simulink model "dinamicaralik"  (R2023b)
settings: Solver=ode45  StartTime=0.0  StopTime=50  FixedStep=0.0001  RelTol=1e-3
InitFcn:
  | Kpz = 0.3 ;
  | KIz = 0;
  | 
  | bh = 0.010290;  % batan hacim m^3
  | m = 10.5     ;  % aracın kütlesi kg
  | g = 9.81     ;  % yer çekimi ivmesi
  | p = 1000     ; % kg / m^3 yogunluk
  | W = m*g      ;  % aracın agırlıgı N
  | B = p*g*bh   ;  % Kaldırma kuvveti  N
  | 
  | xg = 0 ; % rgid body frame e göre ağırlık merkzi kordinatları
  | yg = 0 ;
  | zg = 0.02 ;
  | 
  | Ix = 0.1011 ; % kg *  m ^2
  | Iy = 0.1159 ;
  | Iz = 0.1615 ;
  | 
  | thrustCoefficient = 50/21.5 ;
  | 
  | % Add mass parametreleri
  | Xu_dot = -5.5;   % Surge direction
  | Yv_dot = -12.7;  % Sway direction
  | Zw_dot = -14.57; % Heave direction
  | 
  | Kp_dot = -0.12;  % Roll moment
  | Mq_dot = -0.12;  % Pitch moment
  | Nr_dot = -0.12;  % Yaw moment
  | 
  | % Linear Damping Values (Doğrusal Sönümleme Katsayıları)
  | Xu = -4.03;   % Ns/m
  | Yv = -6.22;   % Ns/m
  | Zw = -5.18;   % Ns/m
  | Kp = -0.07;   % Ns/rad
  | Mq = -0.07;   % Ns/rad
  | Nr = -0.07;   % Ns/rad
  | 
  | % Quadratic Damping Values (Doğrusal Olmayan Sönümleme Katsayıları)
  | Xuu = -18.18;  % Ns^2/m^2
  | Yvv = -21.66;  % Ns^2/m^2
  | Zww = -36.99;  % Ns^2/m^2
  | Kpp = -1.55;   % Ns^2/rad^2
  | Mqq = -1.55;   % Ns^2/rad^2
  | Nrr = -1.55;   % Ns^2/rad^2
undefined symbols (not defined in the file or in its folder): smiData, X, Y, Z
libraries: slpidlib x41, nesl_utility x14, sm_lib x12
(part 1 of 7)
settings Model: Creator=Yaser  LastModifiedBy=User

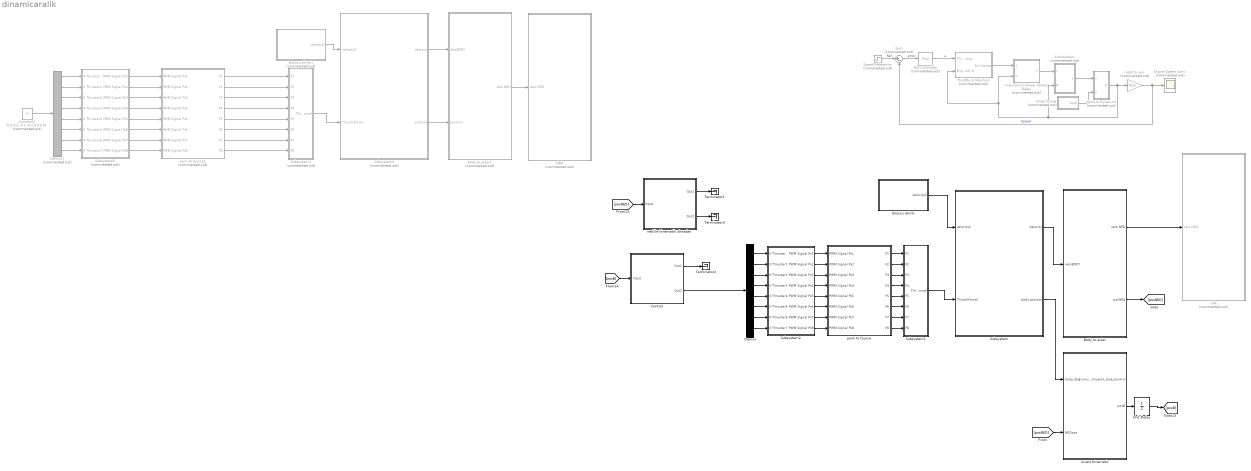
== system dinamicaralik ==
  Body to euler : Subsystem
  Body to euler1 : Subsystem  Commented=on
  Bozucu akıntı : Subsystem
  Bozucu akıntı1 : Subsystem  Commented=on
  Combustion : Subsystem  Commented=on
      settings: RTWMemSecFuncInitTerm=Default  RTWMemSecFuncExecute=Default  RTWMemSecDataConstants=Default  RTWMemSecDataInternal=Default  RTWMemSecDataParameters=Default
  Constant1 : Constant  Commented=on  Value=[0.2 0.2 -0.2 -0.2 0 0 0 0]  VectorParams1D=off
  Control : Subsystem
  Demux : Demux  Outputs=8
  Demux1 : Demux  Commented=on  Outputs=8
  Drag Torque : Subsystem  Commented=on
      settings: RTWMemSecFuncInitTerm=Default  RTWMemSecFuncExecute=Default  RTWMemSecDataConstants=Default  RTWMemSecDataInternal=Default  RTWMemSecDataParameters=Default
  Engine Speed (rpm) : Scope  Commented=on
  Induction to Power Stroke Delay : Subsystem  Commented=on
      settings: RTWMemSecFuncInitTerm=Default  RTWMemSecFuncExecute=Default  RTWMemSecDataConstants=Default  RTWMemSecDataInternal=Default  RTWMemSecDataParameters=Default
  Invers Kinematic : Subsystem
  PID Controller : slpidlib/PID Controller  Commented=on  Controller=PI  Form=Parallel  TimeDomain=Continuous-time  UseExternalTs=off  SampleTime=1  IntegratorMethod=Forward Euler  FilterMethod=Forward Euler  ControllerParametersSource=internal  P=1  I=1  UseKiTs=off  D=0  N=100  UseFilter=on  TunerSelectOption=Transfer Function Based (PID Tuner App)  ZeroCross=off  InitialConditionSource=internal  InitialConditionForIntegrator=8.9768  InitialConditionForFilter=0  DifferentiatorICPrevScaledInput=0  ExternalReset=none  TrackingMode=off  Kt=1  LimitOutput=off  SatLimitsSource=internal  UpperSaturationLimit=inf  LowerSaturationLimit=-inf  LinearizeAsGain=off  AntiWindupMode=none  Kb=1  LimitIntegrator=off  UpperIntegratorSaturationLimit=inf  LowerIntegratorSaturationLimit=-inf  POutMin=[ ]  POutMax=[ ]  IOutMin=[ ]  IOutMax=[ ]  DOutMin=[ ]  DOutMax=[ ]  NOutMin=[ ]  NOutMax=[ ]  SumOutMin=[ ]  SumOutMax=[ ]  SaturationOutMin=[ ]  SaturationOutMax=[ ]  PParamMin=[ ]  PParamMax=[ ]  IParamMin=[ ]  IParamMax=[ ]  DParamMin=[ ]  DParamMax=[ ]  NParamMin=[ ]  NParamMax=[ ]  KbParamMin=[ ]  KbParamMax=[ ]  KtParamMin=[ ]  KtParamMax=[ ]  KbOutMin=[ ]  KbOutMax=[ ]  KtOutMin=[ ]  KtOutMax=[ ]  IntegratorOutMin=[ ]  IntegratorOutMax=[ ]  FilterOutMin=[ ]  FilterOutMax=[ ]  SumI1OutMin=[ ]  SumI1OutMax=[ ]  SumI2OutMin=[ ]  SumI2OutMax=[ ]  SumI3OutMin=[ ]  SumI3OutMax=[ ]  SumI4OutMin=[]  SumI4OutMax=[]  SumDOutMin=[ ]  SumDOutMax=[ ]  DifferentiatorOutMin=[]  DifferentiatorOutMax=[]  FilterDiffOutCoefMin=[]  FilterDiffOutCoefMax=[]  ReciprocalOutMin=[]  ReciprocalOutMax=[]  SumDenOutMin=[]  SumDenOutMax=[]  SumNumOutMin=[]  SumNumOutMax=[]  DivideOutMin=[]  DivideOutMax=[]  UdiffTsProdOutMin=[]  UdiffTsProdOutMax=[]  NTsProdOutMin=[]  NTsProdOutMax=[]  UintegralTsProdOutMin=[]  UintegralTsProdOutMax=[]  UngainTsProdOutMin=[]  UngainTsProdOutMax=[]  ClampingZeroOutDataTypeStr=Inherit: Inherit via back propagation  ClampingZeroOutMin=[]  ClampingZeroOutMax=[]  FilterDenConstantOutDataTypeStr=Inherit: Inherit via back propagation  FilterDenConstantOutMin=[]  FilterDenConstantOutMax=[]  PCopyOutDataTypeStr=Inherit: Inherit via back propagation  PCopyOutMin=[]  PCopyOutMax=[]  NCopyOutDataTypeStr=Inherit: Inherit via back propagation  NCopyOutMin=[]  NCopyOutMax=[]  IntegratorContinuousStateAttributes=''  IntegratorStateMustResolveToSignalObject=off  IntegratorRTWStateStorageClass=Auto  FilterContinuousStateAttributes=''  FilterStateMustResolveToSignalObject=off  FilterRTWStateStorageClass=Auto  ParallelPVariant=InternalParameters  IdealPVariant=Disabled  IVariant=InternalParameters  DVariant=Disabled  IntegratorVariant=Continuous  SatVariant=Disabled  AWVariant=Passthrough  PCopyVariant=Disabled  TRVariant=Disabled  FdbkBlocksVariant=Forward  IdealPFdbkVariant=Disabled  SatFdbkVariant=Disabled  DerivativeFilterVariant=Disabled  NVariant=Disabled  NCopyVariant=Disabled_SignalSpec  FilterICVariant=Disabled  IntegratorICVariant=InternalICs  ExternalResetVariant=Disabled  TRSumVariant=Passthrough  SumFdbkVariant=Disabled  SumVariant=Sum_PI  TsampFilterVariant=InternalTs  TsampNgainVariant=Passthrough  TsampIntegralVariant=Disabled_SignalSpec  ExternalSaturationOutDataTypeStr=Inherit: Same as second input
  Speed Reference : Step  Commented=on  Time=2  Before=2000  After=3000  SampleTime=0
  Subsystem : Subsystem
  Subsystem1 : Subsystem
  Subsystem2 : Subsystem
  Subsystem3 : Subsystem  Commented=on
  Subsystem4 : Subsystem  Commented=on
  Subsystem5 : Subsystem  Commented=on
  Sum : Sum  Commented=on  Inputs=|+-
  SİM : Subsystem  Commented=on
  SİM1 : Subsystem  Commented=on
  Terminator1 : Terminator
  Terminator2 : Terminator
  Terminator3 : Terminator
  Throttle & Manifold : Subsystem  Commented=on
      settings: RTWMemSecFuncInitTerm=Default  RTWMemSecFuncExecute=Default  RTWMemSecDataConstants=Default  RTWMemSecDataInternal=Default  RTWMemSecDataParameters=Default
  Unit Delay : UnitDelay  SampleTime=0.01  HasFrameUpgradeWarning=on
  Vehicle Dynamics : Subsystem  Commented=on
      settings: RTWMemSecFuncInitTerm=Default  RTWMemSecFuncExecute=Default  RTWMemSecDataConstants=Default  RTWMemSecDataInternal=Default  RTWMemSecDataParameters=Default
  ned ile kinematik olmadan : Subsystem
  pwm to fource : Subsystem
  pwm to fource1 : Subsystem  Commented=on
  rad/s to rpm : Gain  Commented=on  Gain=30/pi  SaturateOnIntegerOverflow=on  OutDataTypeStr=Inherit: Same as input  ParamDataTypeStr=Inherit: Same as input
  wires:
  rad/s to rpm/1 -> Engine Speed (rpm)/1, Sum/2  "Speed"
  Throttle & Manifold/1(Air charge) -> Induction to Power Stroke Delay/1(Air charge)
  Induction to Power Stroke Delay/1(Air Charge) -> Combustion/1(Air Charge)
  Vehicle Dynamics/1(N) -> Combustion/2(N), Induction to Power Stroke Delay/2(N), Throttle & Manifold/2("Engine Speed, N"), rad/s to rpm/1
  Sum/1 -> PID Controller/1  "error"
  Combustion/1(Torque) -> Vehicle Dynamics/1(Teng)
  Drag Torque/1(Load) -> Vehicle Dynamics/2(Tload)
  PID Controller/1 -> Throttle & Manifold/1(Throttle Ang.)  "u"
  Speed Reference/1 -> Sum/1  "Ref"
  pwm to fource/4(F4) -> Subsystem1/4(F4)
  pwm to fource/3(F3) -> Subsystem1/3(F3)
  pwm to fource/2(F2) -> Subsystem1/2(F2)
  pwm to fource/1(F1) -> Subsystem1/1(F1)
  pwm to fource/5(F5) -> Subsystem1/5(F5)
  pwm to fource/6(F6) -> Subsystem1/6(F6)
  pwm to fource/7(F7) -> Subsystem1/7(F7)
  pwm to fource/8(F8) -> Subsystem1/8(F8)
  Subsystem2/1(PWM Signal Px1) -> pwm to fource/1(PWM Signal Px1)
  Subsystem2/2(PWM Signal Px2) -> pwm to fource/2(PWM Signal Px2)
  Subsystem2/3(PWM Signal Px3) -> pwm to fource/3(PWM Signal Px3)
  Subsystem2/4(PWM Signal Px4) -> pwm to fource/4(PWM Signal Px4)
  Subsystem2/5(PWM Signal Px5) -> pwm to fource/5(PWM Signal Px5)
  Subsystem2/6(PWM Signal Px6) -> pwm to fource/6(PWM Signal Px6)
  Subsystem2/7(PWM Signal Px7) -> pwm to fource/7(PWM Signal Px7)
  Subsystem2/8(PWM Signal Px8) -> pwm to fource/8(PWM Signal Px8)
  Bozucu akıntı/1(velocityC) -> Subsystem/1(velocityC)
  Subsystem/1(Velocity) -> Body to euler/1(veloBODY)
  Body to euler/1(velo NED) -> SİM/1(velo NED)
  Subsystem1/1(Thrust(Force)) -> Subsystem/2(Thrust(Force))
  Subsystem3/2(position) -> Body to euler1/2(position)
  Body to euler1/1(velo NED) -> SİM1/1(velo NED)
  Bozucu akıntı1/1(velocityC) -> Subsystem3/1(velocityC)
  Subsystem4/1(Thrust(Force)) -> Subsystem3/2(Thrust(Force))
  Subsystem5/6(PWM Signal Px6) -> pwm to fource1/6(PWM Signal Px6)
  Demux1/7 -> Subsystem5/7(X Thruster6)
  Subsystem5/5(PWM Signal Px5) -> pwm to fource1/5(PWM Signal Px5)
  Demux1/4 -> Subsystem5/4(X Thruster3)
  Subsystem5/7(PWM Signal Px7) -> pwm to fource1/7(PWM Signal Px7)
  Constant1/1 -> Demux1/1
  Demux1/2 -> Subsystem5/2(X Thruster1)
  Demux1/5 -> Subsystem5/5(X Thruster4)
  Demux1/1 -> Subsystem5/1(X Thruster)
  Subsystem5/8(PWM Signal Px8) -> pwm to fource1/8(PWM Signal Px8)
  Subsystem5/1(PWM Signal Px1) -> pwm to fource1/1(PWM Signal Px1)
  Demux1/3 -> Subsystem5/3(X Thruster2)
  pwm to fource1/6(F6) -> Subsystem4/6(F6)
  Subsystem3/1(Velocity) -> Body to euler1/1(veloBODY)
  Subsystem5/4(PWM Signal Px4) -> pwm to fource1/4(PWM Signal Px4)
  pwm to fource1/4(F4) -> Subsystem4/4(F4)
  Demux1/6 -> Subsystem5/6(X Thruster5)
  Subsystem5/2(PWM Signal Px2) -> pwm to fource1/2(PWM Signal Px2)
  pwm to fource1/5(F5) -> Subsystem4/5(F5)
  pwm to fource1/8(F8) -> Subsystem4/8(F8)
  pwm to fource1/2(F2) -> Subsystem4/2(F2)
  pwm to fource1/1(F1) -> Subsystem4/1(F1)
  Demux1/8 -> Subsystem5/8(X Thruster7)
  pwm to fource1/3(F3) -> Subsystem4/3(F3)
  pwm to fource1/7(F7) -> Subsystem4/7(F7)
  Subsystem5/3(PWM Signal Px3) -> pwm to fource1/3(PWM Signal Px3)
  Demux/1 -> Subsystem2/1(X Thruster)
  Demux/2 -> Subsystem2/2(X Thruster1)
  Demux/3 -> Subsystem2/3(X Thruster2)
  Demux/4 -> Subsystem2/4(X Thruster3)
  Demux/5 -> Subsystem2/5(X Thruster4)
  Demux/6 -> Subsystem2/6(X Thruster5)
  Demux/7 -> Subsystem2/7(X Thruster6)
  Demux/8 -> Subsystem2/8(X Thruster7)
  Body to euler/2(posNEd) -> [posNED]
  ned ile kinematik olmadan/1(Out1) -> Terminator1/1
  [posNED] -> ned ile kinematik olmadan/1(Input)
  Control/1(Out1) -> Terminator2/1
  Control/2(Out2) -> Demux/1
  [posB] -> Control/1(Input)
  ned ile kinematik olmadan/2(Out2) -> Terminator3/1
  Subsystem/2(body position) -> Invers Kinematic/1(body_doğrumudonuşum_diye_kontrol)
  [posNED] -> Invers Kinematic/2(NEDpos)
  Invers Kinematic/1(posB) -> Unit Delay/1
  Unit Delay/1 -> [posB]

== system dinamicaralik/Body to euler ==
  veloBODY : Inport
  Integrator : Integrator
  To Workspace : ToWorkspace  VariableName=pos  SaveFormat=Timeseries  SampleTime=-1
  euler transform : MATLAB Function  TreatAsAtomicUnit=on
  velo NED : Outport
  posNEd : Outport  Port=2
  wires:
  veloBODY/1 -> euler transform/1(veloB)
  euler transform/1(NEDvelo) -> Integrator/1, velo NED/1
  Integrator/1 -> To Workspace/1, posNEd/1

== system dinamicaralik/Body to euler1 ==
  veloBODY : Inport
  position : Inport  Port=2
  Integrator : Integrator
  To Workspace : ToWorkspace  VariableName=pos  SaveFormat=Timeseries  SampleTime=-1
  euler transform : MATLAB Function  TreatAsAtomicUnit=on
  velo NED : Outport
  wires:
  veloBODY/1 -> euler transform/1(veloB)
  euler transform/1(NEDvelo) -> Integrator/1, velo NED/1
  Integrator/1 -> To Workspace/1

== system dinamicaralik/Bozucu akıntı ==
  Constant : Constant  Value=[0 0 0 0 0 0 ]
  Constant1 : Constant  Commented=on  Value=[0 0 0 0 0 0 ]
  velocityC : Outport
  wires:
  Constant/1 -> velocityC/1

== system dinamicaralik/Bozucu akıntı1 ==
  Constant : Constant  Value=[0 0 0 0 0 0 ]
  Constant1 : Constant  Commented=on  Value=[0 0 0 0 0 0 ]
  velocityC : Outport
  wires:
  Constant/1 -> velocityC/1

== system dinamicaralik/Combustion ==
  note: Engine Torque
  Air Charge : Inport
  N : Inport  Port=2
  Mux : Mux
  Spark Advance : Constant  Value=15.0
  Stoichiometric Fuel : Gain  Gain=1/14.6  SaturateOnIntegerOverflow=on  OutDataTypeStr=Inherit: Same as input  ParamDataTypeStr=Inherit: Same as input
  Sum : Sum  InputSameDT=on  SaturateOnIntegerOverflow=on  OutDataTypeStr=Inherit: Same as first input
  Torque Gen : Fcn  Expr=-181.3 + 379.36*u[1] + 21.91*u[1]/u[2] - (0.85*u[1]*u[1])/(u[2]*u[2]) + 0.26*u[3] - 0.0028*u[3]*u[3]
  Torque Gen2 : Fcn  Expr=0.027*u[4] - 0.000107*u[4]*u[4] + 0.00048*u[4]*u[3] + 2.55*u[3]*u[1] - 0.05*u[3]*u[3]*u[1]
  Torque : Outport  InitialOutput=0  VectorParamsAs1DForOutWhenUnconnected=off
  wires:
  Stoichiometric Fuel/1 -> Mux/2
  Spark Advance/1 -> Mux/3
  N/1 -> Mux/4
  Air Charge/1 -> Stoichiometric Fuel/1, Mux/1
  Mux/1 -> Torque Gen/1, Torque Gen2/1
  Torque Gen2/1 -> Sum/2
  Torque Gen/1 -> Sum/1
  Sum/1 -> Torque/1

== system dinamicaralik/Control ==
  Input : Inport
  From : From  Commented=on  GotoTag=posNED
  divecont : Subsystem  Commented=on
  divecont1 : Subsystem
  Out1 : Outport
  Out2 : Outport  Port=2
  wires:
  Input/1 -> divecont1/1(Input)
  divecont1/1(Out1) -> Out2/1
  divecont/1(Out1) -> Out1/1
  From/1 -> divecont/1(In1)

== system dinamicaralik/Drag Torque ==
  note: Torque Disturbances
  Step : Step  Time=2  Before=25  After=25  SampleTime=0
  Step1 : Step  Time=8  After=0  SampleTime=0
  Sum1 : Sum  InputSameDT=on  SaturateOnIntegerOverflow=on  OutDataTypeStr=Inherit: Same as first input
  Load : Outport  InitialOutput=0  VectorParamsAs1DForOutWhenUnconnected=off
  wires:
  Step1/1 -> Sum1/2
  Step/1 -> Sum1/1
  Sum1/1 -> Load/1

== system dinamicaralik/Induction to Power Stroke Delay ==
  Air charge : Inport
  N : Inport  Port=2
  Constant2 : Constant  Value=pi
  Divide1 : Product  Inputs=/*
  dM/dt delay : VariableTransportDelay  MaximumDelay=10  InitialOutput=0.152  MaximumPoints=10240  TransDelayFeedthrough=on  PadeOrder=2
  Air Charge : Outport  VectorParamsAs1DForOutWhenUnconnected=off
  wires:
  dM/dt delay/1 -> Air Charge/1
  Constant2/1 -> Divide1/2
  N/1 -> Divide1/1
  Divide1/1 -> dM/dt delay/2
  Air charge/1 -> dM/dt delay/1

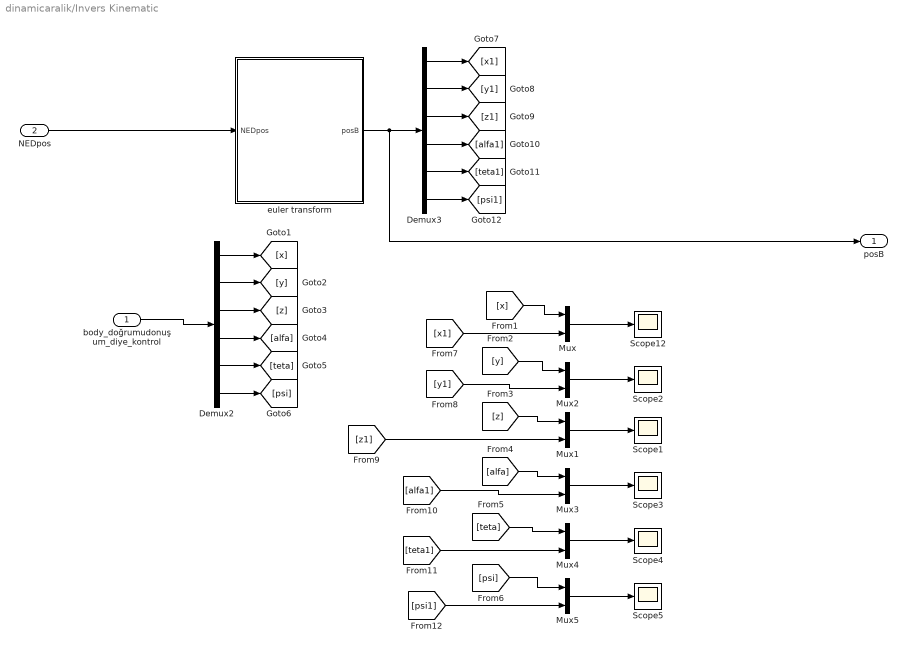
== system dinamicaralik/Invers Kinematic ==
  body_doğrumudonuşum_diye_kontrol : Inport
  NEDpos : Inport  Port=2
  Demux2 : Demux  Outputs=6
  Demux3 : Demux  Outputs=6
  Mux{,1..5} (6 alike) : Mux  Inputs=2
  Scope{1..5,12} (6 alike) : Scope
  euler transform : MATLAB Function  TreatAsAtomicUnit=on
  posB : Outport
  wires:
  [psi1] -> Mux5/2
  body_doğrumudonuşum_diye_kontrol/1 -> Demux2/1
  [x1] -> Mux/2
  Mux4/1 -> Scope4/1
  [z] -> Mux1/1
  euler transform/1(posB) -> posB/1, Demux3/1
  Demux3/1 -> [x1]
  Demux3/4 -> [alfa1]
  Demux3/5 -> [teta1]
  [z1] -> Mux1/2
  [y1] -> Mux2/2
  Mux3/1 -> Scope3/1
  [x] -> Mux/1
  Demux2/5 -> [teta]
  [psi] -> Mux5/1
  Demux3/6 -> [psi1]
  [alfa1] -> Mux3/2
  [teta1] -> Mux4/2
  [alfa] -> Mux3/1
  [teta] -> Mux4/1
  Mux2/1 -> Scope2/1
  Demux3/2 -> [y1]
  Demux2/1 -> [x]
  Mux1/1 -> Scope1/1
  [y] -> Mux2/1
  Demux3/3 -> [z1]
  Demux2/3 -> [z]
  Mux5/1 -> Scope5/1
  NEDpos/1 -> euler transform/1(NEDpos)
  Demux2/2 -> [y]
  Demux2/6 -> [psi]
  Mux/1 -> Scope12/1
  Demux2/4 -> [alfa]

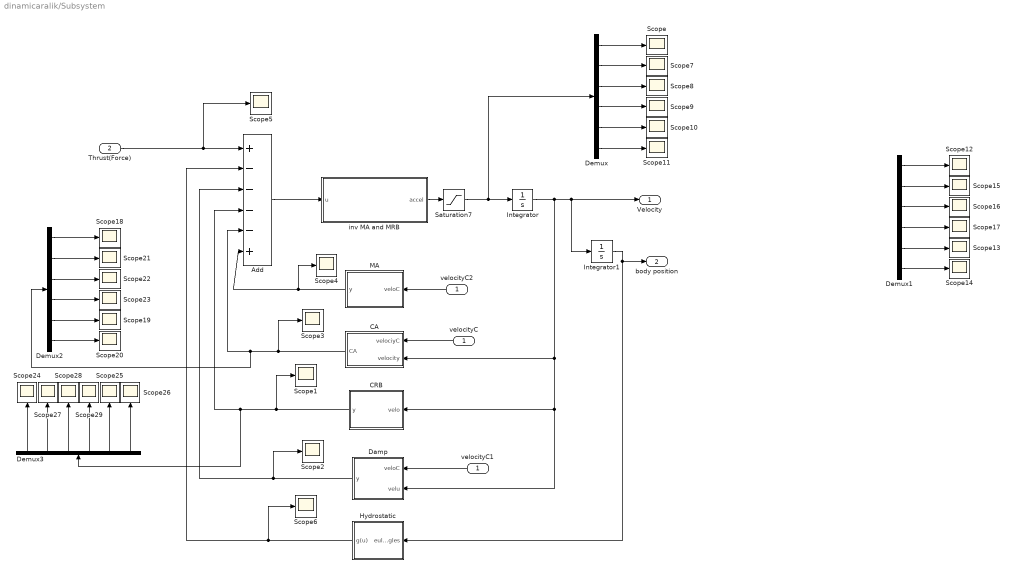
== system dinamicaralik/Subsystem ==
  velocityC : Inport
  Thrust(Force) : Inport  Port=2
  Add : Sum  Inputs=+----+
  CA : Subsystem
  CRB : Subsystem
  Damp : Subsystem
  Demux{,1..3} (4 alike) : Demux  Outputs=6
  Hydrostatic : Subsystem
  Integrator : Integrator
  Integrator1 : Integrator
  MA : Subsystem
  Saturation7 : Saturate  UpperLimit=1000  LowerLimit=-100
  Scope{,1..29} (30 alike) : Scope
  inv MA and MRB : Subsystem
  velocityC1 : InportShadow
  velocityC2 : InportShadow
  Velocity : Outport
  body position : Outport  Port=2
  wires:
  CA/1(CA) -> Scope3/1, Demux2/1, Add/5
  CRB/1(y) -> Scope1/1, Demux3/1, Add/4
  Integrator1/1 -> body position/1, Hydrostatic/1(euler angles)
  Add/1 -> inv MA and MRB/1(u)
  Integrator/1 -> Integrator1/1, Velocity/1, Damp/2(velu), CRB/1(velo), CA/2(velocity)
  Hydrostatic/1(g(u)) -> Scope6/1, Add/2
  Damp/1(y) -> Scope2/1, Add/3
  velocityC/1 -> CA/1(velociyC)
  velocityC1/1 -> Damp/1(veloC)
  velocityC2/1 -> MA/1(veloC)
  MA/1(y) -> Scope4/1, Add/6
  inv MA and MRB/1(accel) -> Saturation7/1
  Saturation7/1 -> Demux/1, Integrator/1
  Thrust(Force)/1 -> Scope5/1, Add/1
  Demux/1 -> Scope/1
  Demux/2 -> Scope7/1
  Demux/3 -> Scope8/1
  Demux/4 -> Scope9/1
  Demux/5 -> Scope10/1
  Demux/6 -> Scope11/1
  Demux1/1 -> Scope12/1
  Demux1/3 -> Scope16/1
  Demux1/6 -> Scope14/1
  Demux1/2 -> Scope15/1
  Demux1/4 -> Scope17/1
  Demux1/5 -> Scope13/1
  Demux2/1 -> Scope18/1
  Demux2/4 -> Scope23/1
  Demux2/2 -> Scope21/1
  Demux2/3 -> Scope22/1
  Demux2/5 -> Scope19/1
  Demux2/6 -> Scope20/1
  Demux3/5 -> Scope25/1
  Demux3/3 -> Scope28/1
  Demux3/2 -> Scope27/1
  Demux3/1 -> Scope24/1
  Demux3/4 -> Scope29/1
  Demux3/6 -> Scope26/1

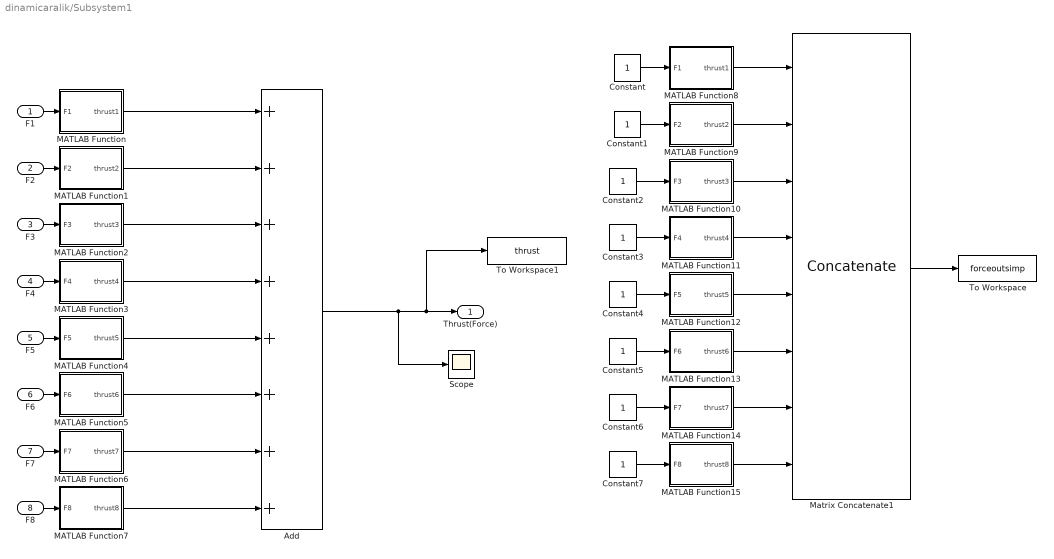
== system dinamicaralik/Subsystem1 ==
  F1 : Inport
  F2 : Inport  Port=2
  F3 : Inport  Port=3
  F4 : Inport  Port=4
  F5 : Inport  Port=5
  F6 : Inport  Port=6
  F7 : Inport  Port=7
  F8 : Inport  Port=8
  Add : Sum  Inputs=++++++++
  Constant{,1..7} (8 alike) : Constant
  MATLAB Function : MATLAB Function  TreatAsAtomicUnit=on
  MATLAB Function1 : MATLAB Function  TreatAsAtomicUnit=on
  MATLAB Function10 : MATLAB Function  TreatAsAtomicUnit=on
  MATLAB Function11 : MATLAB Function  TreatAsAtomicUnit=on
  MATLAB Function12 : MATLAB Function  TreatAsAtomicUnit=on
  MATLAB Function13 : MATLAB Function  TreatAsAtomicUnit=on
  MATLAB Function14 : MATLAB Function  TreatAsAtomicUnit=on
  MATLAB Function15 : MATLAB Function  TreatAsAtomicUnit=on
  MATLAB Function2 : MATLAB Function  TreatAsAtomicUnit=on
  MATLAB Function3 : MATLAB Function  TreatAsAtomicUnit=on
  MATLAB Function4 : MATLAB Function  TreatAsAtomicUnit=on
  MATLAB Function5 : MATLAB Function  TreatAsAtomicUnit=on
  MATLAB Function6 : MATLAB Function  TreatAsAtomicUnit=on
  MATLAB Function7 : MATLAB Function  TreatAsAtomicUnit=on
  MATLAB Function8 : MATLAB Function  TreatAsAtomicUnit=on
  MATLAB Function9 : MATLAB Function  TreatAsAtomicUnit=on
  Matrix Concatenate1 : Concatenate  NumInputs=8  Mode=Multidimensional array  ConcatenateDimension=2
  Scope : Scope
  To Workspace : ToWorkspace  VariableName=forceoutsimp  SaveFormat=Timeseries  SampleTime=-1
  To Workspace1 : ToWorkspace  VariableName=thrust  SaveFormat=Timeseries  SampleTime=-1
  Thrust(Force) : Outport
  wires:
  F1/1 -> MATLAB Function/1(F1)
  F4/1 -> MATLAB Function3/1(F4)
  F7/1 -> MATLAB Function6/1(F7)
  F3/1 -> MATLAB Function2/1(F3)
  F8/1 -> MATLAB Function7/1(F8)
  F5/1 -> MATLAB Function4/1(F5)
  F2/1 -> MATLAB Function1/1(F2)
  F6/1 -> MATLAB Function5/1(F6)
  MATLAB Function/1(thrust1) -> Add/1
  MATLAB Function1/1(thrust2) -> Add/2
  MATLAB Function3/1(thrust4) -> Add/4
  MATLAB Function4/1(thrust5) -> Add/5
  MATLAB Function5/1(thrust6) -> Add/6
  MATLAB Function6/1(thrust7) -> Add/7
  MATLAB Function7/1(thrust8) -> Add/8
  Add/1 -> Scope/1, To Workspace1/1, Thrust(Force)/1
  MATLAB Function2/1(thrust3) -> Add/3
  Constant7/1 -> MATLAB Function15/1(F8)
  Constant5/1 -> MATLAB Function13/1(F6)
  Constant2/1 -> MATLAB Function10/1(F3)
  Constant6/1 -> MATLAB Function14/1(F7)
  Constant/1 -> MATLAB Function8/1(F1)
  Constant4/1 -> MATLAB Function12/1(F5)
  Constant1/1 -> MATLAB Function9/1(F2)
  MATLAB Function14/1(thrust7) -> Matrix Concatenate1/7
  MATLAB Function9/1(thrust2) -> Matrix Concatenate1/2
  MATLAB Function13/1(thrust6) -> Matrix Concatenate1/6
  MATLAB Function8/1(thrust1) -> Matrix Concatenate1/1
  MATLAB Function10/1(thrust3) -> Matrix Concatenate1/3
  MATLAB Function11/1(thrust4) -> Matrix Concatenate1/4
  MATLAB Function15/1(thrust8) -> Matrix Concatenate1/8
  MATLAB Function12/1(thrust5) -> Matrix Concatenate1/5
  Constant3/1 -> MATLAB Function11/1(F4)
  Matrix Concatenate1/1 -> To Workspace/1

== system dinamicaralik/Subsystem2 ==
  X Thruster : Inport
  X Thruster1 : Inport  Port=2
  X Thruster2 : Inport  Port=3
  X Thruster3 : Inport  Port=4
  X Thruster4 : Inport  Port=5
  X Thruster5 : Inport  Port=6
  X Thruster6 : Inport  Port=7
  X Thruster7 : Inport  Port=8
  1-D Lookup Table{,1..7} (8 alike) : Lookup_n-D  NumberOfTableDimensions=1  BreakpointsForDimension1=[-1:0.01:1]  Table=1500 + 400 * ([-1:0.01:1])  InternalRulePriority=Speed  RndMeth=Simplest
  PWM Signal Px1 : Outport
  PWM Signal Px2 : Outport  Port=2
  PWM Signal Px3 : Outport  Port=3
  PWM Signal Px4 : Outport  Port=4
  PWM Signal Px5 : Outport  Port=5
  PWM Signal Px6 : Outport  Port=6
  PWM Signal Px7 : Outport  Port=7
  PWM Signal Px8 : Outport  Port=8
  wires:
  X Thruster2/1 -> 1-D Lookup Table2/1
  X Thruster5/1 -> 1-D Lookup Table5/1
  X Thruster/1 -> 1-D Lookup Table/1
  X Thruster6/1 -> 1-D Lookup Table6/1
  X Thruster4/1 -> 1-D Lookup Table4/1
  X Thruster1/1 -> 1-D Lookup Table1/1
  X Thruster3/1 -> 1-D Lookup Table3/1
  1-D Lookup Table1/1 -> PWM Signal Px2/1
  X Thruster7/1 -> 1-D Lookup Table7/1
  1-D Lookup Table/1 -> PWM Signal Px1/1
  1-D Lookup Table7/1 -> PWM Signal Px8/1
  1-D Lookup Table2/1 -> PWM Signal Px3/1
  1-D Lookup Table6/1 -> PWM Signal Px7/1
  1-D Lookup Table3/1 -> PWM Signal Px4/1
  1-D Lookup Table5/1 -> PWM Signal Px6/1
  1-D Lookup Table4/1 -> PWM Signal Px5/1

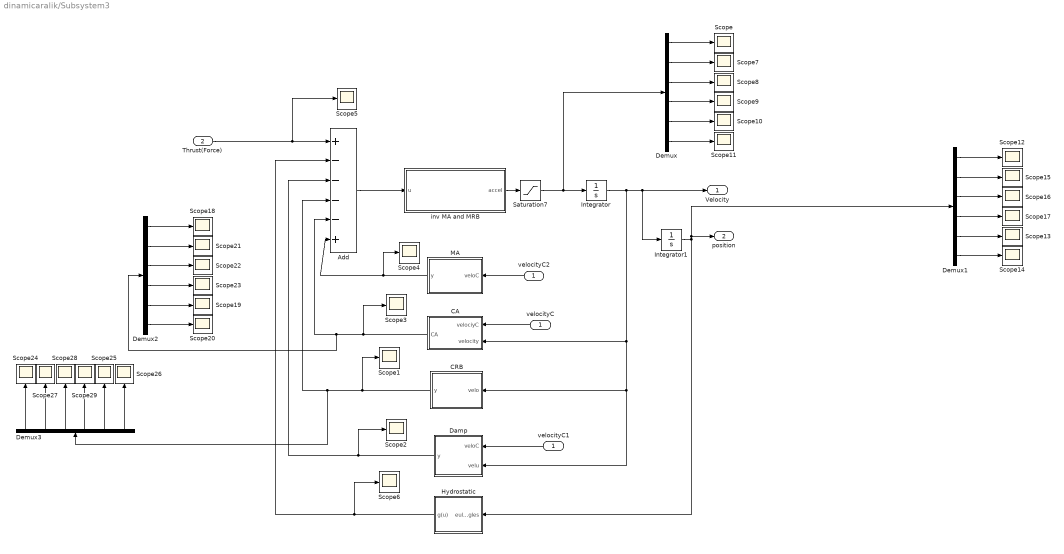
== system dinamicaralik/Subsystem3 ==
  velocityC : Inport
  Thrust(Force) : Inport  Port=2
  Add : Sum  Inputs=+----+
  CA : Subsystem
  CRB : Subsystem
  Damp : Subsystem
  Demux{,1..3} (4 alike) : Demux  Outputs=6
  Hydrostatic : Subsystem
  Integrator : Integrator
  Integrator1 : Integrator
  MA : Subsystem
  Saturation7 : Saturate  UpperLimit=1000  LowerLimit=-100
  Scope{,1..29} (30 alike) : Scope
  inv MA and MRB : Subsystem
  velocityC1 : InportShadow
  velocityC2 : InportShadow
  Velocity : Outport
  position : Outport  Port=2
  wires:
  CA/1(CA) -> Scope3/1, Demux2/1, Add/5
  CRB/1(y) -> Scope1/1, Demux3/1, Add/4
  Integrator1/1 -> Demux1/1, position/1, Hydrostatic/1(euler angles)
  Add/1 -> inv MA and MRB/1(u)
  Integrator/1 -> Integrator1/1, Velocity/1, Damp/2(velu), CRB/1(velo), CA/2(velocity)
  Hydrostatic/1(g(u)) -> Scope6/1, Add/2
  Damp/1(y) -> Scope2/1, Add/3
  velocityC/1 -> CA/1(velociyC)
  velocityC1/1 -> Damp/1(veloC)
  velocityC2/1 -> MA/1(veloC)
  MA/1(y) -> Scope4/1, Add/6
  inv MA and MRB/1(accel) -> Saturation7/1
  Saturation7/1 -> Demux/1, Integrator/1
  Thrust(Force)/1 -> Scope5/1, Add/1
  Demux/1 -> Scope/1
  Demux/2 -> Scope7/1
  Demux/3 -> Scope8/1
  Demux/4 -> Scope9/1
  Demux/5 -> Scope10/1
  Demux/6 -> Scope11/1
  Demux1/1 -> Scope12/1
  Demux1/3 -> Scope16/1
  Demux1/6 -> Scope14/1
  Demux1/2 -> Scope15/1
  Demux1/4 -> Scope17/1
  Demux1/5 -> Scope13/1
  Demux2/1 -> Scope18/1
  Demux2/4 -> Scope23/1
  Demux2/2 -> Scope21/1
  Demux2/3 -> Scope22/1
  Demux2/5 -> Scope19/1
  Demux2/6 -> Scope20/1
  Demux3/5 -> Scope25/1
  Demux3/3 -> Scope28/1
  Demux3/2 -> Scope27/1
  Demux3/1 -> Scope24/1
  Demux3/4 -> Scope29/1
  Demux3/6 -> Scope26/1

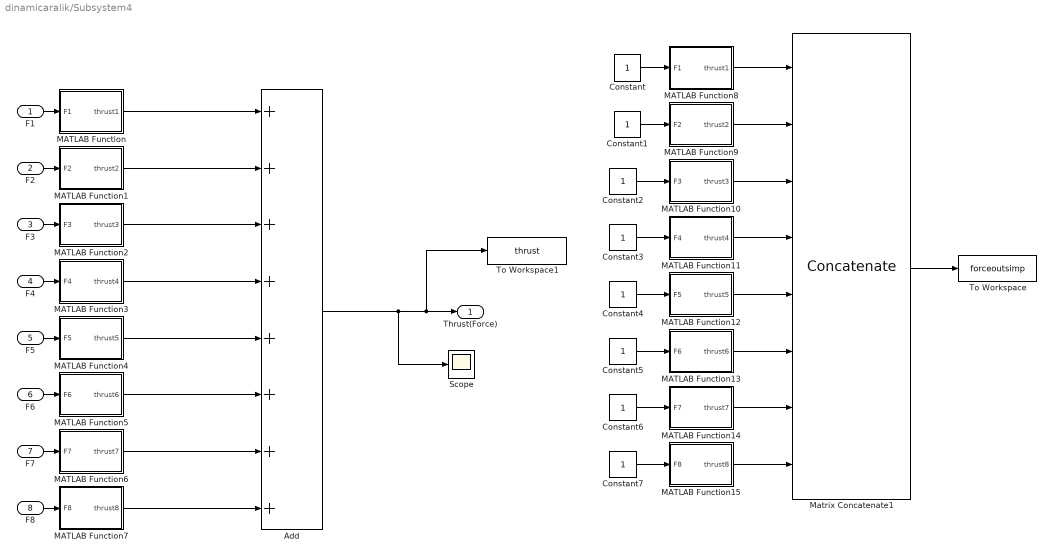
== system dinamicaralik/Subsystem4 ==
  F1 : Inport
  F2 : Inport  Port=2
  F3 : Inport  Port=3
  F4 : Inport  Port=4
  F5 : Inport  Port=5
  F6 : Inport  Port=6
  F7 : Inport  Port=7
  F8 : Inport  Port=8
  Add : Sum  Inputs=++++++++
  Constant{,1..7} (8 alike) : Constant
  MATLAB Function : MATLAB Function  TreatAsAtomicUnit=on
  MATLAB Function1 : MATLAB Function  TreatAsAtomicUnit=on
  MATLAB Function10 : MATLAB Function  TreatAsAtomicUnit=on
  MATLAB Function11 : MATLAB Function  TreatAsAtomicUnit=on
  MATLAB Function12 : MATLAB Function  TreatAsAtomicUnit=on
  MATLAB Function13 : MATLAB Function  TreatAsAtomicUnit=on
  MATLAB Function14 : MATLAB Function  TreatAsAtomicUnit=on
  MATLAB Function15 : MATLAB Function  TreatAsAtomicUnit=on
  MATLAB Function2 : MATLAB Function  TreatAsAtomicUnit=on
  MATLAB Function3 : MATLAB Function  TreatAsAtomicUnit=on
  MATLAB Function4 : MATLAB Function  TreatAsAtomicUnit=on
  MATLAB Function5 : MATLAB Function  TreatAsAtomicUnit=on
  MATLAB Function6 : MATLAB Function  TreatAsAtomicUnit=on
  MATLAB Function7 : MATLAB Function  TreatAsAtomicUnit=on
  MATLAB Function8 : MATLAB Function  TreatAsAtomicUnit=on
  MATLAB Function9 : MATLAB Function  TreatAsAtomicUnit=on
  Matrix Concatenate1 : Concatenate  NumInputs=8  Mode=Multidimensional array  ConcatenateDimension=2
  Scope : Scope
  To Workspace : ToWorkspace  VariableName=forceoutsimp  SaveFormat=Timeseries  SampleTime=-1
  To Workspace1 : ToWorkspace  VariableName=thrust  SaveFormat=Timeseries  SampleTime=-1
  Thrust(Force) : Outport
  wires:
  F1/1 -> MATLAB Function/1(F1)
  F4/1 -> MATLAB Function3/1(F4)
  F7/1 -> MATLAB Function6/1(F7)
  F3/1 -> MATLAB Function2/1(F3)
  F8/1 -> MATLAB Function7/1(F8)
  F5/1 -> MATLAB Function4/1(F5)
  F2/1 -> MATLAB Function1/1(F2)
  F6/1 -> MATLAB Function5/1(F6)
  MATLAB Function/1(thrust1) -> Add/1
  MATLAB Function1/1(thrust2) -> Add/2
  MATLAB Function3/1(thrust4) -> Add/4
  MATLAB Function4/1(thrust5) -> Add/5
  MATLAB Function5/1(thrust6) -> Add/6
  MATLAB Function6/1(thrust7) -> Add/7
  MATLAB Function7/1(thrust8) -> Add/8
  Add/1 -> Scope/1, To Workspace1/1, Thrust(Force)/1
  MATLAB Function2/1(thrust3) -> Add/3
  Constant7/1 -> MATLAB Function15/1(F8)
  Constant5/1 -> MATLAB Function13/1(F6)
  Constant2/1 -> MATLAB Function10/1(F3)
  Constant6/1 -> MATLAB Function14/1(F7)
  Constant/1 -> MATLAB Function8/1(F1)
  Constant4/1 -> MATLAB Function12/1(F5)
  Constant1/1 -> MATLAB Function9/1(F2)
  MATLAB Function14/1(thrust7) -> Matrix Concatenate1/7
  MATLAB Function9/1(thrust2) -> Matrix Concatenate1/2
  MATLAB Function13/1(thrust6) -> Matrix Concatenate1/6
  MATLAB Function8/1(thrust1) -> Matrix Concatenate1/1
  MATLAB Function10/1(thrust3) -> Matrix Concatenate1/3
  MATLAB Function11/1(thrust4) -> Matrix Concatenate1/4
  MATLAB Function15/1(thrust8) -> Matrix Concatenate1/8
  MATLAB Function12/1(thrust5) -> Matrix Concatenate1/5
  Constant3/1 -> MATLAB Function11/1(F4)
  Matrix Concatenate1/1 -> To Workspace/1

== system dinamicaralik/Subsystem5 ==
  X Thruster : Inport
  X Thruster1 : Inport  Port=2
  X Thruster2 : Inport  Port=3
  X Thruster3 : Inport  Port=4
  X Thruster4 : Inport  Port=5
  X Thruster5 : Inport  Port=6
  X Thruster6 : Inport  Port=7
  X Thruster7 : Inport  Port=8
  1-D Lookup Table{,1..7} (8 alike) : Lookup_n-D  NumberOfTableDimensions=1  BreakpointsForDimension1=[-1:0.01:1]  Table=1500 + 400 * ([-1:0.01:1])  InternalRulePriority=Speed  RndMeth=Simplest
  PWM Signal Px1 : Outport
  PWM Signal Px2 : Outport  Port=2
  PWM Signal Px3 : Outport  Port=3
  PWM Signal Px4 : Outport  Port=4
  PWM Signal Px5 : Outport  Port=5
  PWM Signal Px6 : Outport  Port=6
  PWM Signal Px7 : Outport  Port=7
  PWM Signal Px8 : Outport  Port=8
  wires:
  X Thruster2/1 -> 1-D Lookup Table2/1
  X Thruster5/1 -> 1-D Lookup Table5/1
  X Thruster/1 -> 1-D Lookup Table/1
  X Thruster6/1 -> 1-D Lookup Table6/1
  X Thruster4/1 -> 1-D Lookup Table4/1
  X Thruster1/1 -> 1-D Lookup Table1/1
  X Thruster3/1 -> 1-D Lookup Table3/1
  1-D Lookup Table1/1 -> PWM Signal Px2/1
  X Thruster7/1 -> 1-D Lookup Table7/1
  1-D Lookup Table/1 -> PWM Signal Px1/1
  1-D Lookup Table7/1 -> PWM Signal Px8/1
  1-D Lookup Table2/1 -> PWM Signal Px3/1
  1-D Lookup Table6/1 -> PWM Signal Px7/1
  1-D Lookup Table3/1 -> PWM Signal Px4/1
  1-D Lookup Table5/1 -> PWM Signal Px6/1
  1-D Lookup Table4/1 -> PWM Signal Px5/1

== system dinamicaralik/SİM ==
  velo NED : Inport
  6-DOF Joint : sm_lib/Joints/6-DOF Joint  JointMode=Normal  SenseConstraintForce=off  SenseConstraintForceX=off  SenseConstraintForceY=off  SenseConstraintForceZ=off  SenseConstraintTorque=off  SenseConstraintTorqueX=off  SenseConstraintTorqueY=off  SenseConstraintTorqueZ=off  SenseTotalForce=off  SenseTotalForceX=off  SenseTotalForceY=off  SenseTotalForceZ=off  SenseTotalTorque=off  SenseTotalTorqueX=off  SenseTotalTorqueY=off  SenseTotalTorqueZ=off  CompositeWrenchDir=FollowerOnBase  CompositeWrenchFrame=BaseFrame  PxEquilibriumPosition=0  PxEquilibriumPositionUnits=m  PxSpringStiffness=0  PxSpringStiffnessUnits=N/m  PxDampingCoefficient=0  PxDampingCoefficientUnits=N/(m/s)  PxTorqueActuationMode=ComputedTorque  PxMotionActuationMode=InputMotion  PxSensePosition=off  PxSenseVelocity=off  PxSenseAcceleration=off  PxSenseTorqueForce=off  PxSenseLowerLimitTorqueForce=off  PxSenseUpperLimitTorqueForce=off  PxLowerLimitSpecify=off  PxLowerLimitBound=-1  PxLowerLimitBoundUnits=m  PxLowerLimitStiffness=1e6  PxLowerLimitStiffnessUnits=N/m  PxLowerLimitDamping=1e3  PxLowerLimitDampingUnits=N/(m/s)  PxLowerLimitTransitionRegionWidth=1e-4  PxLowerLimitTransitionRegionWidthUnits=m  PxUpperLimitSpecify=off  PxUpperLimitBound=1  PxUpperLimitBoundUnits=m  PxUpperLimitStiffness=1e6  PxUpperLimitStiffnessUnits=N/m  PxUpperLimitDamping=1e3  PxUpperLimitDampingUnits=N/(m/s)  PxUpperLimitTransitionRegionWidth=1e-4  PxUpperLimitTransitionRegionWidthUnits=m  PxPositionTargetSpecify=off  PxPositionTargetPriority=High  PxPositionTargetValue=0  PxPositionTargetValueUnits=m  PxVelocityTargetSpecify=off  PxVelocityTargetPriority=High  PxVelocityTargetValue=0  PxVelocityTargetValueUnits=m/s  PyEquilibriumPosition=0  PyEquilibriumPositionUnits=m  PySpringStiffness=0  PySpringStiffnessUnits=N/m  PyDampingCoefficient=0  PyDampingCoefficientUnits=N/(m/s)  PyTorqueActuationMode=ComputedTorque  PyMotionActuationMode=InputMotion  PySensePosition=off  PySenseVelocity=off  PySenseAcceleration=off  PySenseTorqueForce=off  PySenseLowerLimitTorqueForce=off  PySenseUpperLimitTorqueForce=off  PyLowerLimitSpecify=off  PyLowerLimitBound=-1  PyLowerLimitBoundUnits=m  PyLowerLimitStiffness=1e6  PyLowerLimitStiffnessUnits=N/m  PyLowerLimitDamping=1e3  PyLowerLimitDampingUnits=N/(m/s)  PyLowerLimitTransitionRegionWidth=1e-4  PyLowerLimitTransitionRegionWidthUnits=m  PyUpperLimitSpecify=off  PyUpperLimitBound=1  PyUpperLimitBoundUnits=m  PyUpperLimitStiffness=1e6  PyUpperLimitStiffnessUnits=N/m  PyUpperLimitDamping=1e3  PyUpperLimitDampingUnits=N/(m/s)  PyUpperLimitTransitionRegionWidth=1e-4  PyUpperLimitTransitionRegionWidthUnits=m  PyPositionTargetSpecify=off  PyPositionTargetPriority=High  PyPositionTargetValue=0  PyPositionTargetValueUnits=m  PyVelocityTargetSpecify=off  PyVelocityTargetPriority=High  PyVelocityTargetValue=0  PyVelocityTargetValueUnits=m/s  PzEquilibriumPosition=0  PzEquilibriumPositionUnits=m  PzSpringStiffness=0  PzSpringStiffnessUnits=N/m  PzDampingCoefficient=0  PzDampingCoefficientUnits=N/(m/s)  PzTorqueActuationMode=ComputedTorque  PzMotionActuationMode=InputMotion  PzSensePosition=off  PzSenseVelocity=off  PzSenseAcceleration=off  PzSenseTorqueForce=off  PzSenseLowerLimitTorqueForce=off  PzSenseUpperLimitTorqueForce=off  PzLowerLimitSpecify=off  PzLowerLimitBound=-1  PzLowerLimitBoundUnits=m  PzLowerLimitStiffness=1e6  PzLowerLimitStiffnessUnits=N/m  PzLowerLimitDamping=1e3  PzLowerLimitDampingUnits=N/(m/s)  PzLowerLimitTransitionRegionWidth=1e-4  PzLowerLimitTransitionRegionWidthUnits=m  PzUpperLimitSpecify=off  PzUpperLimitBound=1  PzUpperLimitBoundUnits=m  PzUpperLimitStiffness=1e6  PzUpperLimitStiffnessUnits=N/m  PzUpperLimitDamping=1e3  PzUpperLimitDampingUnits=N/(m/s)  PzUpperLimitTransitionRegionWidth=1e-4  PzUpperLimitTransitionRegionWidthUnits=m  PzPositionTargetSpecify=off  PzPositionTargetPriority=High  PzPositionTargetValue=0  PzPositionTargetValueUnits=m  PzVelocityTargetSpecify=off  PzVelocityTargetPriority=High  PzVelocityTargetValue=0  PzVelocityTargetValueUnits=m/s  SphEqPosRotationMethod=None  SphEqPosRotationAngleUnits=deg  SphEqPosRotationStandardAxis=+Z  SphEqPosRotationAngle=0  SphEqPosRotationArbitraryAxis=[0 0 1]  SphEqPosFollAlignAxisA=+X  SphEqPosBaseAlignAxisA=+Y  SphEqPosFollAlignAxisB=+Y  SphEqPosBaseAlignAxisB=+Z  SphEqPosRotationSequenceAxes=FollowerAxes  SphEqPosRotationSequence=XYX  SphEqPosRotationSequenceAngles=[0 0 0]  SphEqPosRotationSequenceAnglesUnits=deg  SphEqPosRotationMatrix=[1 0 0;0 1 0;0 0 1]  SphEqPosQuaternion=[1 0 0 0]  SphSpringStiffness=0  SphSpringStiffnessUnits=N*m/deg  SphDampingCoefficient=0  SphDampingCoefficientUnits=N*m/(deg/s)  SphActuateTorqueX=on  SphActuateTorqueY=on  SphActuateTorqueZ=on  SphActuateTorque=off  SphTorqueActuationMode=InputTorque  SphMotionActuationMode=ComputedMotion  SphActuationFrame=BaseFrame  SphSensePosition=off  SphSenseVelocityX=off  SphSenseVelocityY=off  SphSenseVelocityZ=off  SphSenseVelocity=off  SphSenseAccelerationX=off  SphSenseAccelerationY=off  SphSenseAccelerationZ=off  SphSenseAcceleration=off  SphSenseTorqueX=off  SphSenseTorqueY=off  SphSenseTorqueZ=off  SphSenseTorqueForce=off  SphSenseLowerLimitTorqueMag=off  SphSenseUpperLimitTorqueMag=off  SphSensingFrame=BaseFrame  SphLowerLimitSpecify=off  SphLowerLimitBound=15  SphLowerLimitBoundUnits=deg  SphLowerLimitStiffness=1e4  SphLowerLimitStiffnessUnits=N*m/deg  SphLowerLimitDamping=10  SphLowerLimitDampingUnits=N*m/(deg/s)  SphLowerLimitTransitionRegionWidth=0.1  SphLowerLimitTransitionRegionWidthUnits=deg  SphUpperLimitSpecify=off  SphUpperLimitBound=45  SphUpperLimitBoundUnits=deg  SphUpperLimitStiffness=1e4  SphUpperLimitStiffnessUnits=N*m/deg  SphUpperLimitDamping=10  SphUpperLimitDampingUnits=N*m/(deg/s)  SphUpperLimitTransitionRegionWidth=0.1  SphUpperLimitTransitionRegionWidthUnits=deg  SphPositionTargetRotationMethod=None  SphPositionTargetRotationAngleUnits=deg  SphPositionTargetRotationStandardAxis=+Z  SphPositionTargetRotationAngle=0  SphPositionTargetRotationArbitraryAxis=[0 0 1]  SphPositionTargetFollAlignAxisA=+X  SphPositionTargetBaseAlignAxisA=+Y  SphPositionTargetFollAlignAxisB=+Y  SphPositionTargetBaseAlignAxisB=+Z  SphPositionTargetRotationSequenceAxes=FollowerAxes  SphPositionTargetRotationSequence=XYX  SphPositionTargetRotationSequenceAngles=[0 0 0]  SphPositionTargetRotationSequenceAnglesUnits=deg  SphPositionTargetRotationMatrix=[1 0 0;0 1 0;0 0 1]  SphPositionTargetQuaternion=[1 0 0 0]  SphPositionTargetSpecify=off  SphPositionTargetPriority=High  SphVelocityTargetValue=[0 0 0]  SphVelocityTargetValueUnits=deg/s  SphVelocityTargetSpecify=off  SphVelocityTargetPriority=High  SphVelocityTargetInFollowerFrame=on
  Cylindrical Solid : sm_lib/Body Elements/Cylindrical Solid  GraphicAmbientColor=[0.15 0.15 0.15 1.0]  BasedOnType=Density  CenterOfMass=[0 0 0]  CenterOfMassUnits=m  GraphicDiffuseColor=[0.5 0.5 0.5]  CylinderLength=1  CylinderLengthUnits=m  CylinderRadius=1  CylinderRadiusUnits=m  Density=1000  DensityUnits=kg/m^3  DoExposeReferenceFrame=on  GraphicEmissiveColor=[0.0 0.0 0.0 1.0]  ExportEntireGeometry=off  SerializedFrames=<Frames/>  MarkerShape=Sphere  MarkerSize=10  GraphicType=FromGeometry  InertiaType=CalculateFromGeometry  Mass=1  MassUnits=kg  MomentsOfInertia=[1 1 1]  MomentsOfInertiaUnits=kg*m^2  GraphicOpacity=1.0  ProductsOfInertia=[0 0 0]  ProductsOfInertiaUnits=kg*m^2  GraphicShininess=75  GraphicSpecularColor=[0.5 0.5 0.5 1.0]  GraphicVisPropType=SimpleVisualProperties
  Demux : Demux  Outputs=6
  Integrator : Integrator
  MechanismConfiguration : sm_lib/Utilities/Mechanism Configuration  UniformGravity=Constant  GravityVector=[0 -9.8 0]  GravityVectorUnits=m/s^2  LinearizationDelta=0.001  JointModeTransitionNonlinearIterations=2
  Simulink-PS Converter{,1..5} (6 alike) : nesl_utility/Simulink-PS Converter  PhysicalDomain=network_engine_domain  SubClassName=ps_input  LeftPortType=input  RightPortType=output  PseudoPeriodic=off  Frequencies=[]  NoiseDistribution=none  NoiseParameters=[]  Unit=1  AffineConversion=off  FilteringAndDerivatives=provide  SimscapeFilterOrder=1  InputFilterTimeConstant=0.001  UdotUserProvided=0
  Solver Configuration : nesl_utility/Solver Configuration  PhysicalDomain=network_engine_domain  SubClassName=solver  LeftPortType=input  RightPortType=generic  Tones=[]  Harmonics=[]  SimulateNoise=off  Profile=off  UseLocalSampling=off  EnableSwitchedLinearOptims=on  FrequencyDomain=off  UseCCode=off  RelTol=0.001  AbsTol=0.001  MinStep=1e-09  ToWorkspace=off  RevertToSquareIcSolve=off  NumHomotopyIterations=100  PhasorMode=off  PhasorModeNumHarmonics=1  ConsistencySolver=NEWTON_XTOL_AFTER_FTOL  IndexReductionMethod=DerivativeReplacement  DoDC=off  ResidualTolerance=1e-09  ConsistencyTolSource=GLOBAL  ConsistencyAbsTol=0.001  ConsistencyRelTol=0.001  ConsistencyTolFactor=0.001  UseLocalSolver=off  LocalSolverChoice=NE_BACKWARD_EULER_ADVANCER  ResolveIndetEquations=on  FunctionEvalNumThread=1  LocalSolverSampleTime=0.001  DoFixedCost=off  MaxNonlinIter=3  MaxModeIter=2  ComputeImpulses=off  ImpulseIterations=2  LinearAlgebra=auto  LinearAlgebraNumThread=0  EquationFormulation=NE_TIME_EF  DelaysMemoryBudget=1024  AutomaticFiltering=on  FilteringTimeConstant=0.001  PartitionStorageMethod=AS_NEEDED  PartitionMemoryBudget=1024  PartitionMethod=ROBUST  MultibodyUseLocalSolver=off  MultibodyLocalSolverChoice=ODE1  MultibodyLocalSolverSampleTime=0.001
  Transform : sm_lib/Frames and Transforms/Rigid Transform  TranslationMethod=Cartesian  TranslationStandardOffset=0  TranslationStandardOffsetUnits=m  TranslationStandardAxis=+Z  TranslationCartesianOffset=smiData.RigidTransform(37).translation  TranslationCartesianOffsetUnits=mm  TranslationROffset=0  TranslationROffsetUnits=m  TranslationZOffset=0  TranslationZOffsetUnits=m  TranslationThetaOffset=0  TranslationThetaOffsetUnits=deg  RotationMethod=ArbitraryAxis  RotationAngleUnits=rad  RotationStandardAxis=+Z  RotationAngle=0  RotationArbitraryAxis=[0,0,0]  FollAlignAxisA=+X  BaseAlignAxisA=+Y  FollAlignAxisB=+Y  BaseAlignAxisB=+Z  RotationSequenceAxes=FollowerAxes  RotationSequence=XYX  RotationSequenceAngles=[0 0 0]  RotationSequenceAnglesUnits=deg  RotationMatrix=[1 0 0;0 1 0;0 0 1]  Quaternion=[1 0 0 0]
  Transform1 : sm_lib/Frames and Transforms/Rigid Transform  TranslationMethod=Cartesian  TranslationStandardOffset=0  TranslationStandardOffsetUnits=m  TranslationStandardAxis=+Z  TranslationCartesianOffset=smiData.RigidTransform(37).translation  TranslationCartesianOffsetUnits=mm  TranslationROffset=0  TranslationROffsetUnits=m  TranslationZOffset=0  TranslationZOffsetUnits=m  TranslationThetaOffset=0  TranslationThetaOffsetUnits=deg  RotationMethod=ArbitraryAxis  RotationAngleUnits=rad  RotationStandardAxis=+Z  RotationAngle=0  RotationArbitraryAxis=[0,0,0]  FollAlignAxisA=+X  BaseAlignAxisA=+Y  FollAlignAxisB=+Y  BaseAlignAxisB=+Z  RotationSequenceAxes=FollowerAxes  RotationSequence=XYX  RotationSequenceAngles=[0 0 0]  RotationSequenceAnglesUnits=deg  RotationMatrix=[1 0 0;0 1 0;0 0 1]  Quaternion=[1 0 0 0]
  World : sm_lib/Frames and Transforms/World Frame
  wires:
  velo NED/1 -> Integrator/1
  Integrator/1 -> Demux/1
  Demux/1 -> Simulink-PS Converter/1
  Demux/2 -> Simulink-PS Converter1/1
  Demux/3 -> Simulink-PS Converter2/1
  Demux/4 -> Simulink-PS Converter3/1
  Demux/5 -> Simulink-PS Converter4/1
  Demux/6 -> Simulink-PS Converter5/1
  connections:
  Solver Configuration/RConn1 -- Transform/LConn1 -- MechanismConfiguration/RConn1 -- World/RConn1
  Simulink-PS Converter/RConn1 -- 6-DOF Joint/LConn2
  Simulink-PS Converter1/RConn1 -- 6-DOF Joint/LConn3
  6-DOF Joint/LConn5 -- Simulink-PS Converter3/RConn1
  6-DOF Joint/LConn4 -- Simulink-PS Converter2/RConn1
  Simulink-PS Converter5/RConn1 -- 6-DOF Joint/LConn7
  Simulink-PS Converter4/RConn1 -- 6-DOF Joint/LConn6
  Transform/RConn1 -- 6-DOF Joint/LConn1
  Transform1/RConn1 -- Cylindrical Solid/RConn1
  6-DOF Joint/RConn1 -- Transform1/LConn1
